simulink model "ActiveSuspensions"  (R2020b)
settings: Solver=VariableStepAuto  StartTime=0.0  StopTime=10.0  MaxStep=0.001  RelTol=1e-3
values from neighbouring files (symbols this model uses):
  x0 = [0.01 ... (first row only)    [Main.m]    (also in SweepTest.m = [- g*ms/ks + l0s + Lift/ks; myActiveSuspensions.mat = [0.597040517241 0 0.3385371843 0 0])
  xeq = -inv(A)*B3*[ls; lt; g]    [Main.m]
settings Model: Creator=nicol  LastModifiedBy=nicol

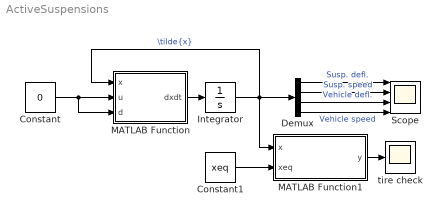
== system ActiveSuspensions ==
  Constant : Constant  Value=0
  Constant1 : Constant  Value=xeq
  Demux : Demux
  Integrator : Integrator  InitialCondition=x0
  MATLAB Function : MATLAB Function  TreatAsAtomicUnit=on
  MATLAB Function1 : MATLAB Function  TreatAsAtomicUnit=on
  Scope : Scope  NumInputPorts=4
  tire check : Scope
  wires:
  Integrator/1 -> MATLAB Function1/1(x), Demux/1, MATLAB Function/1(x)  "\\tilde{x}"
  MATLAB Function/1(dxdt) -> Integrator/1
  Constant/1 -> MATLAB Function/3(d), MATLAB Function/2(u)
  Demux/1 -> Scope/1  "Susp. defl."
  Demux/2 -> Scope/2  "Susp. speed"
  Demux/3 -> Scope/3  "Vehicle defl."
  Demux/4 -> Scope/4  "Vehicle speed"
  MATLAB Function1/1(y) -> tire check/1
  Constant1/1 -> MATLAB Function1/2(xeq)

== matlab function ActiveSuspensions/MATLAB Function ==
  data: x input; u input; dxdt output; d input
function dxdt = Plant(x,u,d)

kt = 160000; % [N/m] tire stiffness

mu = 25; % [kg] unsprung mass
ms = 300; % [kg] sprung mass
barm = 1/mu + 1/ms; % [1/kg]

betas = 1000; % [N/(m/s)]  damping coeff.
ks = 16000; % [N/m] suspension stiffness

A = [ 0 1  0 0
     -ks*barm-kt/mu -betas*barm kt/mu 0
     0 0 0 1
     -ks/ms -betas/ms 0 0];
 
B1 = [0
     barm
     0
     1/ms];

 B2 = [0
     0
     0
     -1];

dxdt = A*x+B1*u+B2*d;

== matlab function ActiveSuspensions/MATLAB Function1 ==
  data: x input; y output; xeq input
function y = TireCheck(x,xeq)

lt = 0.05; % [m] tire unloaded length

tildex3 = x(3);
tildex1 = x(1);

x3eq = xeq(3);
x1eq = xeq(1);


y = tildex3-tildex1-(lt-x3eq+x1eq);
